simulink model "rlPlaysSnake"  (R2021a)
settings: Solver=VariableStepAuto  StartTime=0.0  StopTime=1000  RelTol=1e-3
model workspace (MAT data in the model file):
  appleBoardInit = 0
  snakeBoardInit = 0
libraries: rllib x1
settings Model: Creator=Mitch  LastModifiedBy=Mitch

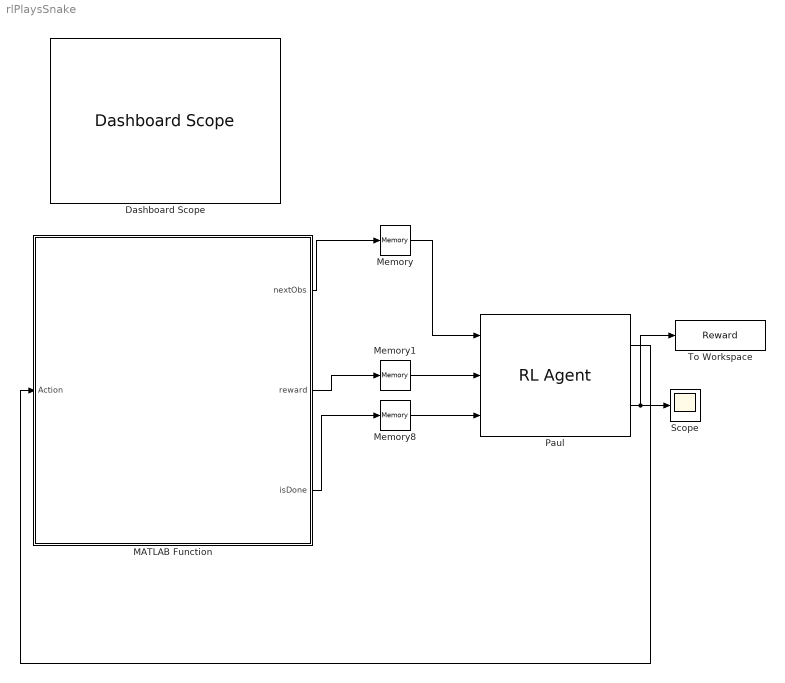
== system rlPlaysSnake ==
  Dashboard Scope : DashboardScope
  MATLAB Function : MATLAB Function  TreatAsAtomicUnit=on
  Memory : Memory
  Memory1 : Memory
  Memory8 : Memory
  Paul : rllib/RL Agent  Agent=Paul  ExternalActionAsInput=off  ProvideCumRwd=on  TreatAsDirectFeedthrough=on
  Scope : Scope
  To Workspace : ToWorkspace  VariableName=Reward  SaveFormat=Timeseries  SampleTime=-1
  wires:
  Paul/2 -> To Workspace/1, Scope/1
  Paul/1 -> MATLAB Function/1(Action)
  Memory1/1 -> Paul/2
  MATLAB Function/3(isDone) -> Memory8/1
  MATLAB Function/2(reward) -> Memory1/1
  Memory8/1 -> Paul/3
  MATLAB Function/1(nextObs) -> Memory/1
  Memory/1 -> Paul/1

== matlab function rlPlaysSnake/MATLAB Function ==
  data: Action input; nextObs output; reward output; isDone output
% function [nextObs, reward, count, snakeBoard, appleLoc, isDone, snakeHead, snakeTail, snakeLength] = ...
%     playGame(Action, count, snakeBoard, appleLoc, snakeHead, snakeTail, snakeLength)

function [nextObs, reward, isDone] = playGame(Action)

reward = 0;

persistent count previousMove;
persistent snakeBoard appleLoc snakeHead snakeTail snakeLength;

BoardSize = 10;
gameBoard = zeros(BoardSize);

if(isempty(previousMove))
    previousMove = 0;
end

if(isempty(count))
    count = 0;
end

if(isempty(appleLoc))
    appleLoc = [3 , 3];
end

if(isempty(snakeHead))
    snakeHead = [5, 5];
end

if(isempty(snakeTail))
    snakeTail = [5, 4];
end

if(isempty(snakeLength))
    snakeLength = 2;
end

if(isempty(snakeBoard))
    snakeBoard = gameBoard;
end


if(count == 0)
    snakeBoard = gameBoard;
    snakeBoard(snakeHead(2), snakeHead(1)) = 1;
    snakeBoard(snakeTail(2), snakeTail(1)) = snakeLength;
    
    score = 0;
    
end
% imshow(combinedBoard)

% imagesc(gameBoard)
% title("Score: " + score)

% Action = input("Pick a Direction [N, E, S, W]");

%Perform Action
switch(Action)
    case(1) %N
        newHeadLoc =  snakeHead + [0, 1];
    case(2) %E
        newHeadLoc =  snakeHead + [1, 0];
    case(3) %S
        newHeadLoc =  snakeHead + [0, -1];
    case(4) %W
        newHeadLoc =  snakeHead + [-1, 0];
    otherwise
        newHeadLoc = [0,0];
        fprintf("\nMake a move")
end

%Evaluate other conditions

if(newHeadLoc == appleLoc)%Hit Apple
    reward = reward + 5;
    isDone = 0;
    
    [~, translation] = lookAround(snakeBoard, snakeTail, "searchValue", snakeLength - 1);
    
    snakeBoard(snakeTail(2) + translation(2), snakeTail(1) + translation(1)) = snakeLength;
    
    snakeLength = snakeLength + 1;
    snakeBoard(snakeTail(2), snakeTail(1)) = snakeLength;
    
    newTailLoc = snakeTail;
    
    appleLoc = randi(BoardSize, [1,2]);
else
    isDone = 0;
    reward = reward + 0;
    
    disp(snakeBoard)
    
    [~, translation] = lookAround(snakeBoard, snakeTail, "searchValue", snakeLength - 1);
    
    snakeBoard(snakeTail(2) + translation(2), snakeTail(1) + translation(1)) = snakeLength;
    
    snakeBoard(snakeTail(2), snakeTail(1)) = 0;
    
    newTailLoc = [snakeTail(1) + translation(1), snakeTail(2) + translation(2)];
end

if((sum(newHeadLoc >= BoardSize) >= 1) || (sum( newHeadLoc <= 0) >= 1))%Hit Wall
    isDone = 1;
    reward = reward - 10;
end

switch(previousMove)
    case(1)
        if(Action == 3)
            isDone = 1;
            Reward = reward - 10;
        end
    case(2)
        if(Action == 4)
            isDone = 1;
            Reward = reward - 10;
        end
    case(3)
        if(Action == 1)
            isDone = 1;
            Reward = reward - 10;
        end
    case(4)
        if(Action == 2)
            isDone = 1;
            Reward = reward - 10;
        end
end

if(isDone == 0)
    if(snakeBoard(newHeadLoc(2), newHeadLoc(1)) ~= 0)%Hit itself
        isDone = 1;
        reward = reward - 10;
    else
        snakeBoard(newHeadLoc(2), newHeadLoc(1)) = 1;
        reward = reward + 1;
    end
end



distanceToApple = real(getDistance(newHeadLoc, appleLoc));

if(isDone == 0)
    if((sum(ismember(gameBoard, 0)) >= 1))
        isDone = 0;
        reward = reward + 1;
    else
        isDone = 1;
        reward = reward + 100;
    end
end

%Adjust All the other values
if(isDone == 0)
    searchNumber = 1;
    startPoint = newHeadLoc;
    while(searchNumber ~= snakeLength)
        [~, translation] = lookAround(snakeBoard, startPoint, "searchvalue", searchNumber);
        if(translation == [0,0])
            break;
        end
        
        startPoint = startPoint + translation;
        
        searchNumber = searchNumber + 1;
        
        snakeBoard(startPoint(2), startPoint(1)) = searchNumber;
        
    end
end

combinedBoard = gameBoard + snakeBoard;

clc
disp(combinedBoard)
pause(1)

previousMove = Action;

nextObs = distanceToApple;
snakeHead = newHeadLoc;
snakeTail = newTailLoc;

count = count + 1;
end
